simulink model "cppControllerMonitor"  (Simulink 8.0)
settings: Solver=FixedStepDiscrete  StartTime=0.0  StopTime=inf  FixedStep=0.01  RelTol=1e-3
libraries: WBCLibrary x2
settings Model: Creator=makaveli  LastModifiedBy=icub

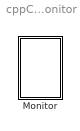
== system cppControllerMonitor ==
  Monitor : Subsystem  mask{moduleName='torqueBalancing', modulePeriod=1}
      mask prompts: moduleName "module name"; modulePeriod "module period"

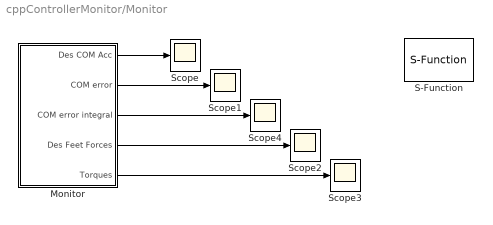
== system cppControllerMonitor/Monitor ==
  Monitor : Subsystem
  S-Function : WBCLibrary/Utilities/S-Function  rate=0.010
  Scope{,1..4} (5 alike) : Scope
      Scope1 settings: YMin=-0.1  YMax=0.6
      Scope2 settings: SaveName=ScopeData2
      Scope3 settings: SaveName=ScopeData3
      Scope4 settings: SaveName=ScopeData4
  wires:
  Monitor/1(Des COM Acc) -> Scope/1
  Monitor/4(Des Feet Forces) -> Scope2/1
  Monitor/5(Torques) -> Scope3/1
  Monitor/2(COM error) -> Scope1/1
  Monitor/3(COM error integral) -> Scope4/1

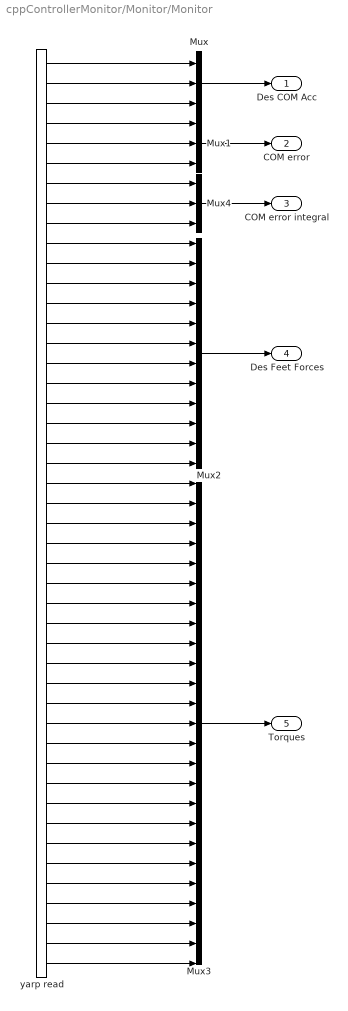
== system cppControllerMonitor/Monitor/Monitor ==
  Mux : Mux  Inputs=3
  Mux1 : Mux  Inputs=3
  Mux2 : Mux  Inputs=12
  Mux3 : Mux  Inputs=25
  Mux4 : Mux  Inputs=3
  yarp read : WBCLibrary/Utilities/yarp read  from=['/' moduleName '/monitor:o']  to='...'  num=46
  Des COM Acc : Outport
  COM error : Outport  Port=2
  COM error integral : Outport  Port=3
  Des Feet Forces : Outport  Port=4
  Torques : Outport  Port=5
  wires:
  yarp read/5 -> Mux1/2
  Mux/1 -> Des COM Acc/1
  Mux2/1 -> Des Feet Forces/1
  Mux1/1 -> COM error/1
  Mux3/1 -> Torques/1
  yarp read/1 -> Mux/1
  yarp read/2 -> Mux/2
  yarp read/4 -> Mux1/1
  yarp read/6 -> Mux1/3
  yarp read/3 -> Mux/3
  Mux4/1 -> COM error integral/1
  yarp read/7 -> Mux4/1
  yarp read/8 -> Mux4/2
  yarp read/9 -> Mux4/3
  yarp read/10 -> Mux2/1
  yarp read/11 -> Mux2/2
  yarp read/12 -> Mux2/3
  yarp read/13 -> Mux2/4
  yarp read/14 -> Mux2/5
  yarp read/15 -> Mux2/6
  yarp read/16 -> Mux2/7
  yarp read/17 -> Mux2/8
  yarp read/18 -> Mux2/9
  yarp read/19 -> Mux2/10
  yarp read/20 -> Mux2/11
  yarp read/21 -> Mux2/12
  yarp read/29 -> Mux3/8
  yarp read/30 -> Mux3/9
  yarp read/31 -> Mux3/10
  yarp read/32 -> Mux3/11
  yarp read/33 -> Mux3/12
  yarp read/34 -> Mux3/13
  yarp read/22 -> Mux3/1
  yarp read/44 -> Mux3/23
  yarp read/45 -> Mux3/24
  yarp read/39 -> Mux3/18
  yarp read/40 -> Mux3/19
  yarp read/35 -> Mux3/14
  yarp read/36 -> Mux3/15
  yarp read/37 -> Mux3/16
  yarp read/43 -> Mux3/22
  yarp read/41 -> Mux3/20
  yarp read/42 -> Mux3/21
  yarp read/38 -> Mux3/17
  yarp read/46 -> Mux3/25
  yarp read/23 -> Mux3/2
  yarp read/24 -> Mux3/3
  yarp read/25 -> Mux3/4
  yarp read/26 -> Mux3/5
  yarp read/27 -> Mux3/6
  yarp read/28 -> Mux3/7
